simulink model "Power_Control"  (R2018a)
settings: Solver=VariableStepAuto  StartTime=0.0  StopTime=10.0  RelTol=1e-3
settings Model: Creator=shami  LastModifiedBy=shami

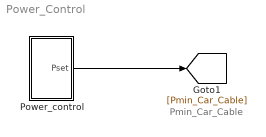
== system Power_Control ==
  note: Pmin_Car_Cable
  Power_control : Subsystem
  wires:
  Power_control/1(Pset) -> [Pmin_Car_Cable]

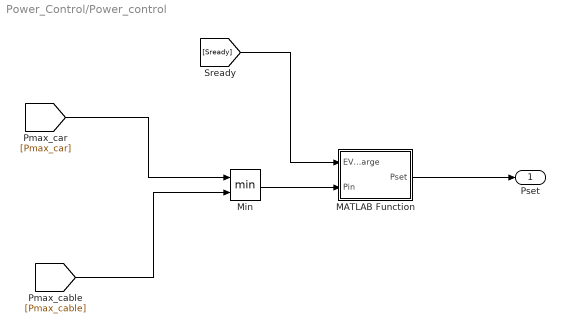
== system Power_Control/Power_control ==
  MATLAB Function : MATLAB Function  TreatAsAtomicUnit=on
  Min : MinMax  Inputs=2
  Pset : Outport
  wires:
  [Pmax_car] -> Min/1
  Min/1 -> MATLAB Function/2(Pin)
  [Pmax_cable] -> Min/2
  MATLAB Function/1(Pset) -> Pset/1
  [Sready] -> MATLAB Function/1(EV_charge)

== matlab function Power_Control/Power_control/MATLAB Function ==
  data: EV_charge input; Pset output; Pin input
function Pset = fcn(EV_charge, Pin)
if EV_charge == 1
    Pset = Pin;
else
    Pset = 0;
end
